simulink model "bask"  (Simulink 6.4)
settings: Solver=FixedStepDiscrete  StartTime=0.0  StopTime=20  RelTol=1e-3
libraries: commsink2 x4, commdigbbndpm3 x3, commchan3 x1, commrandsrc2 x1
settings Model: Creator=ALEX  LastModifiedBy=student
settings OptimizationCC: InitFltsAndDblsToZero=off
settings DebuggingCC: SignalResolutionControl=UseLocalSettings  MultiTaskDSMMsg=error  MultiTaskCondExecSysMsg=error
settings GRTTargetCC: TargetFcnLib=ansi_tfl_table_tmw.mat

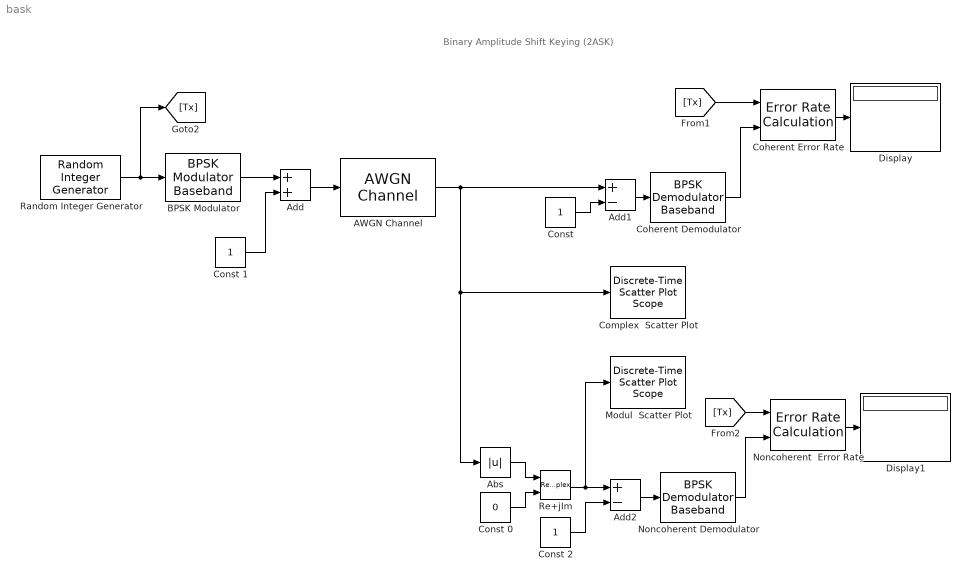
== system bask ==
  note: Binary Amplitude Shift Keying (2ASK)
  AWGN Channel : commchan3/AWGN Channel  SystemSampleTime=-1  seed=67  noiseMode="Signal to noise ratio  (Es/No)"  EbNodB=3  EsNodB=100  SNRdB=10  bitsPerSym=1  Ps=2  Tsym=1  variance=0.2
  Abs : Abs  SampleTime=-1  SaturateOnIntegerOverflow=off
  Add : Sum  OutDataType=fixdt(1, 16)  OutScaling=2^-10
  Add1 : Sum  Inputs=+-  OutDataType=fixdt(1, 16)  OutScaling=2^-10
  Add2 : Sum  Inputs=+-  OutDataType=fixdt(1, 16)  OutScaling=2^-10
  BPSK Modulator : commdigbbndpm3/BPSK Modulator Baseband  SystemSampleTime=-1  Ph=0  outDtype=double  outWordLen=16  outUDDataType=sfix(16)  outFracLenMode=Best precision  outFracLen=15
  "Coherent Demodulator " : commdigbbndpm3/BPSK Demodulator Baseband  SystemSampleTime=-1  Ph=0  outDtype=double
  Coherent Error Rate : commsink2/Error Rate Calculation  N=0  st_delay=0  cp_mode=Entire frame  subframe=[]  PMode=Port  WsName=ErrorVec  RsMode2=off  stop=off  numErr=10000  maxBits=100000
  Complex  Scatter Plot : commsink2/Discrete-Time Scatter Plot Scope  Tag=ScatterPlot  SystemSampleTime=-1  sampPerSymb=1  offsetEye=0  numTraces=100  numNewFrames=10  LineMarkers=.  LineColors=b  fading=on  render=on  AxisGrid=on  xMin=-3.3  xMax=3.315  yMin=-3.3  yMax=3.315  inphaseLabel=In-phase Amplitude  quadratureLabel=Quadrature Amplitude  openScopeAtSimStart=off  FrameNumber=off  FigPos=[360 435 560 487]  figTitle=Scatter Plot  numLinesMax=8  block_type_=scatter
  "Const " : Constant  Value=1  OutDataType=fixdt(1, 16)  ConRadixGroup=Use specified scaling  OutScaling=2^0  SampleTime=inf  FramePeriod=inf
  Const 0 : Constant  Value=0  OutDataType=fixdt(1, 16)  ConRadixGroup=Use specified scaling  OutScaling=2^0  SampleTime=inf  FramePeriod=inf
  Const 1 : Constant  Value=1  OutDataType=fixdt(1, 16)  ConRadixGroup=Use specified scaling  OutScaling=2^0  SampleTime=inf  FramePeriod=inf
  Const 2 : Constant  Value=1  OutDataType=fixdt(1, 16)  ConRadixGroup=Use specified scaling  OutScaling=2^0  SampleTime=inf  FramePeriod=inf
  Display : Display
  Display1 : Display
  Modul  Scatter Plot : commsink2/Discrete-Time Scatter Plot Scope  Tag=ScatterPlot  SystemSampleTime=-1  sampPerSymb=1  offsetEye=0  numTraces=100  numNewFrames=10  LineMarkers=.  LineColors=b  fading=on  render=on  AxisGrid=on  xMin=-3.3  xMax=3.315  yMin=-3.3  yMax=3.315  inphaseLabel=In-phase Amplitude  quadratureLabel=Quadrature Amplitude  openScopeAtSimStart=off  FrameNumber=off  FigPos=[360 435 560 487]  figTitle=Scatter Plot  numLinesMax=8  block_type_=scatter
  "Noncoherent Demodulator " : commdigbbndpm3/BPSK Demodulator Baseband  SystemSampleTime=-1  Ph=0  outDtype=double
  Noncoherent  Error Rate : commsink2/Error Rate Calculation  N=0  st_delay=0  cp_mode=Entire frame  subframe=[]  PMode=Port  WsName=ErrorVec  RsMode2=off  stop=on  numErr=10000  maxBits=100000
  Random Integer Generator : commrandsrc2/Random Integer Generator  SystemSampleTime=-1  mul=2  seed=37  Ts=1  frameBased=off  sampPerFrame=8  orient=off  outDataType=double
  Re+jIm : RealImagToComplex
  wires:
  Random Integer Generator/1 -> BPSK Modulator/1, [Tx]
  Coherent Error Rate/1 -> Display/1
  Const 1/1 -> Add/2
  BPSK Modulator/1 -> Add/1
  Add/1 -> AWGN Channel/1
  Abs/1 -> Re+jIm/1
  Add1/1 -> "Coherent Demodulator "/1
  AWGN Channel/1 -> Abs/1, Complex  Scatter Plot/1, Add1/1
  "Coherent Demodulator "/1 -> Coherent Error Rate/2
  Const 0/1 -> Re+jIm/2
  "Const "/1 -> Add1/2
  [Tx] -> Coherent Error Rate/1
  [Tx] -> Noncoherent  Error Rate/1
  Add2/1 -> "Noncoherent Demodulator "/1
  Re+jIm/1 -> Add2/1, Modul  Scatter Plot/1
  "Noncoherent Demodulator "/1 -> Noncoherent  Error Rate/2
  Noncoherent  Error Rate/1 -> Display1/1
  Const 2/1 -> Add2/2
